simulink model "lab10_sim"  (R2021a)
settings: Solver=ode4  StartTime=0.0  StopTime=20  FixedStep=0.01  RelTol=1e-3
values from neighbouring files (symbols this model uses):
  A = [0 0 0; 1 0 -1; 0 1 2]    [lab10.m]
  B = [0 -1; 1 0; 0 1]    [lab10.m]
  C = [1, 0, 1]    [lab10.m]
  F = F0 + g * f_T    [alocare.m]    (also in lab10.m = alocare(A, B, Lambda_d))
settings Model: Creator=Administrator  LastModifiedBy=Administrator

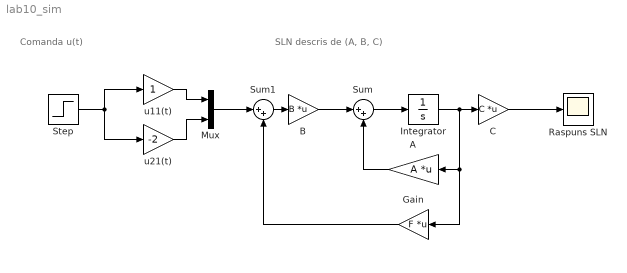
== system lab10_sim ==
  note: SLN descris de (A, B, C)
  note: Comanda u(t)
  A : Gain  Gain=A  Multiplication=Matrix(K*u)
  B : Gain  Gain=B  Multiplication=Matrix(K*u)
  C : Gain  Gain=C  Multiplication=Matrix(K*u)
  Gain : Gain  Gain=F  Multiplication=Matrix(K*u)
  Integrator : Integrator
  Mux : Mux  Inputs=2
  Raspuns SLN : Scope
  Step : Step  SampleTime=0
  Sum : Sum  Inputs=|++
  Sum1 : Sum  Inputs=|++
  u11(t) : Gain
  u21(t) : Gain  Gain=-2
  wires:
  Step/1 -> u21(t)/1, u11(t)/1
  u11(t)/1 -> Mux/1
  u21(t)/1 -> Mux/2
  B/1 -> Sum/1
  Sum/1 -> Integrator/1
  A/1 -> Sum/2
  Integrator/1 -> Gain/1, A/1, C/1
  C/1 -> Raspuns SLN/1
  Mux/1 -> Sum1/1
  Gain/1 -> Sum1/2
  Sum1/1 -> B/1
